simulink model "dc_motor_5hp_model1"  (R2022a)
settings: Solver=ode45  StartTime=0.0  StopTime=6  RelTol=1e-3  EnableMultiTasking=on
values from neighbouring files (symbols this model uses):
  Dm = 1e-4    (= 0.0001)    [dc_par.m]    (also in dcm_par.m = 6.04e-06)
  J = 1    [dc_par.m]    (also in dcm_par.m = 2.12e-06)
  Laf = 1.8    [dc_par.m]    (also in dcm_par.m = 0.0395)
  Ra = 0.6    [dc_par.m]    (also in dcm_par.m = 7)
  Rf = 240    [dc_par.m]
  Ta = La/Ra    (= 0.02)    [dc_par.m]    (also in dcm_par.m = 0.0171428571429)
  Tf = Lf/Rf    (= 0.5)    [dc_par.m]
  Tm = 29    [dc_par.m]    (also in dcm_par.m = 0.00353)
  Va = 240    [dc_par.m]    (also in dcm_par.m = 6)
settings Model: Creator=Jurij  LastModifiedBy=Juri
settings SolverCC: AlgebraicLoopSolver=TrustRegion
settings DataIOCC: LimitDataPoints=on  MaxDataPoints=10000  SaveFormat=Array  SignalLoggingSaveFormat=ModelDataLogs  SaveOutput=off  SaveState=on  ReturnWorkspaceOutputs=off  StateSaveName=x  TimeSaveName=t  SignalLoggingName=sigsOut
settings OptimizationCC: LifeSpan=inf
settings DebuggingCC: SaveWithParameterizedLinksMsg=none  UnderspecifiedInitializationDetection=Classic  MergeDetectMultiDrivingBlocksExec=none  SignalResolutionControl=TryResolveAllWithWarning  MultiTaskDSMMsg=warning  MultiTaskCondExecSysMsg=none  UnconnectedInputMsg=warning  UnconnectedOutputMsg=warning  UnconnectedLineMsg=warning  SFUnexpectedBacktrackingDiag=warning  SFNoUnconditionalDefaultTransitionDiag=warning  SFExecutionAtInitializationDiag=none  SFMachineParentedDataDiag=warning  ArithmeticOperatorsInVariantConditions=warning
settings HardwareCC: ProdBitPerPointer=32  ProdBitPerSizeT=32  ProdBitPerPtrDiffT=32  ProdLargestAtomicFloat=None  ProdIntDivRoundTo=Undefined  ProdEndianess=Unspecified  ProdWordSize=32  ProdHWDeviceType=32-bit Generic  TargetUnknown=on
settings ModelReferenceCC: PropagateSignalLabelsOutOfModel=off
settings SFSimCC: SimUseLocalCustomCode=off  CustomCodeUndefinedFunction=UseInterfaceOnly
settings RTWCC: RTWUseLocalCustomCode=off
settings CodeAppCC: StateflowObjectComments=on
settings GRTTargetCC: TargetLangStandard=C89/C90 (ANSI)  CombineOutputUpdateFcns=off  GRTInterface=on
settings ConfigComp: CovMetricSettings=dw  CovSaveCumulativeToWorkspaceVar=on  CovSaveSingleToWorkspaceVar=on  CovExternalEMLEnable=off

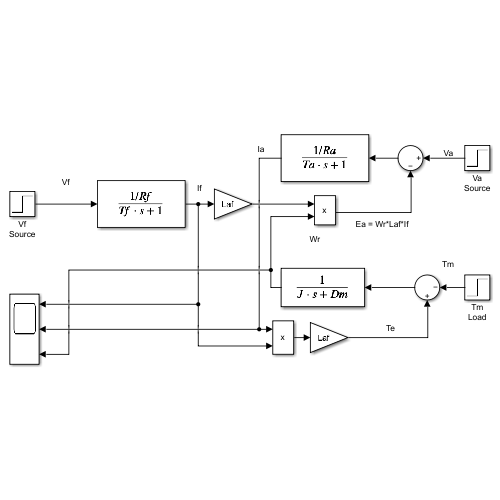
[thumbnail: Simulink's stored preview of the top-level diagram]
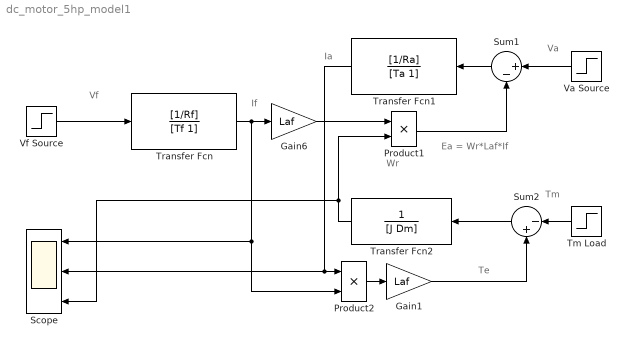
== system dc_motor_5hp_model1 ==
  note: Ia
  note: If
  note: Ea = Wr*Laf*If
  note: Wr
  note: Te
  note: Tm
  note: Va
  note: Vf
  Gain1 : Gain  Gain=Laf  SaturateOnIntegerOverflow=on  OutDataTypeStr=Inherit: Same as input  ParamDataTypeStr=Inherit: Same as input
  Gain6 : Gain  Gain=Laf  SaturateOnIntegerOverflow=on  OutDataTypeStr=Inherit: Same as input  ParamDataTypeStr=Inherit: Same as input
  Product1 : Product  SaturateOnIntegerOverflow=on  OutDataTypeStr=Inherit: Same as first input
  Product2 : Product  SaturateOnIntegerOverflow=on  OutDataTypeStr=Inherit: Same as first input
  Scope : Scope  NumInputPorts=3
  Sum1 : Sum  Inputs=|+-  SaturateOnIntegerOverflow=on
  Sum2 : Sum  Inputs=|-+  SaturateOnIntegerOverflow=on
  Tm Load : Step  Time=4  After=Tm  SampleTime=0
  Transfer Fcn : TransferFcn  Numerator=[1/Rf]  Denominator=[Tf 1]
  Transfer Fcn1 : TransferFcn  Numerator=[1/Ra]  Denominator=[Ta 1]
  Transfer Fcn2 : TransferFcn  Denominator=[J Dm]
  Va Source : Step  Time=2  After=Va  SampleTime=0
  Vf Source : Step  Time=0  Before=Va  After=Va  SampleTime=0
  wires:
  Transfer Fcn/1 -> Gain6/1, Product2/2, Scope/1
  Gain6/1 -> Product1/1
  Sum1/1 -> Transfer Fcn1/1
  Va Source/1 -> Sum1/1
  Vf Source/1 -> Transfer Fcn/1
  Transfer Fcn2/1 -> Product1/2, Scope/3
  Product1/1 -> Sum1/2
  Sum2/1 -> Transfer Fcn2/1
  Tm Load/1 -> Sum2/1
  Product2/1 -> Gain1/1
  Transfer Fcn1/1 -> Product2/1, Scope/2
  Gain1/1 -> Sum2/2
